simulink model "Noa_Nofusion"  (R2020b)
settings: Solver=FixedStepDiscrete  StartTime=0.0  StopTime=Inf  FixedStep=0.01  RelTol=1e-3
PostLoadFcn:
  | if any(exist('dsrtsu_mdlpostloadfcn', 'file') ~= 0), dsrtsu_mdlpostloadfcn('Execute', bdroot); end
InitFcn:
  | , if any(exist('rtifpga_mdlclblib', 'file') ~= 0), rtifpga_mdlclblib('Init', bdroot); end,
  | , if any(exist('dsmpb_private', 'file') ~= 0), dsmpb_private('dsmpb_mdlclblib', 'Init', bdroot); end,
undefined symbols (not defined in the file or in its folder): ACC_TimeGap_DecSetSwt, ACC_TimeGap_IncSetSwt, AccelPedalPosn, AccelPedalPosnVldty, AccelPedlPosnDiagc, AccPedalOverride, ACU_ShiftInProgress, ADAS_Posn_CurLane, AESSwtReq, ALC_SwtReq, BrkPedalSts, CC_ACC_CANCEL_OFFSwt, CC_ACC_CRUISE_OFFSwt, CC_ACC_DecSetSpd_SetSwt, CC_ACC_IncSetSpd_ResuSwt, CC_ACCSwtErr, CharSpd_ms, CSA_NODE, CURRENT_GEAR, CurrentGearValid, DiscIntNeverNeededParam, DrvDoorSts, DrvSBR, DrvTrqReqOvld, ECMACCInterface, ECMRespACC, ELKSwtReq, EngLimpHomeSts, EngSpd, EngState, EngState_PHEV, EngTrqMaxActSpd, EngTrqMinAct, EPS_DrvInpTrqVal_HighReslolution, EPS_FailSts, EPS_LKATorqOvrlDlvd, EPS_LKATorqOvrlDlvdVld, EPS_LKATrqOvlDlvdSts, EPS_SteerMod, EPS_TrqSnsrSts, EQ4_APPINFO, EQ4_LA_ELEM, EQ4_LA_HDR, EQ4_LAP_ELEM, EQ4_LAP_HDR, EQ4_LH_ELEM, EQ4_LH_HDR, EQ4_LRE_ELEM, EQ4_LRE_HDR, ESS_PedSwtReq, ESS_VehSwtReq, FFogLmpSts_F_Pbox, FLWheelDriveDirection, FLWheelSpd, FrntWiprSwtSts, FrntWshrSwtSts, FRWheelDriveDirection, FRWheelSpd, HazardLmpSwtSts, HCU_AccelPedalPosn_Diag ... (+151)
libraries: simulink x144, dsmpblib x33, canfdmsglib x10
(part 6 of 20)

== system Noa_Nofusion/CR_RSDS_Input/RSDS_R_Bus ==
  Enable : EnablePort
  Bus Creator : BusCreator  Inputs=9
  Bus Selector : BusSelector  OutputSignals=RSDS_R_Obj1.RSDS_R_ObjID_1 Value,RSDS_R_Obj2.RSDS_R_ObjID_2 Value,RSDS_R_Obj3.RSDS_R_ObjID_3 Value,RSDS_R_Obj4.RSDS_R_ObjID_4 Value,RSDS_R_Obj5.RSDS_R_ObjID_5 Value,RSDS_R_Obj6.RSDS_R_ObjID_6 Value
  Bus Selector1 : BusSelector  OutputSignals=RSDS_R_Obj1.RSDS_R_ObjDistX_1 Value,RSDS_R_Obj2.RSDS_R_ObjDistX_2 Value,RSDS_R_Obj3.RSDS_R_ObjDistX_3 Value,RSDS_R_Obj4.RSDS_R_ObjDistX_4 Value,RSDS_R_Obj5.RSDS_R_ObjDistX_5 Value,RSDS_R_Obj6.RSDS_R_ObjDistX_6 Value
  Bus Selector2 : BusSelector  OutputSignals=RSDS_R_Obj1.RSDS_R_ObjDistY_1 Value,RSDS_R_Obj2.RSDS_R_ObjDistY_2 Value,RSDS_R_Obj3.RSDS_R_ObjDistY_3 Value,RSDS_R_Obj4.RSDS_R_ObjDistY_4 Value,RSDS_R_Obj5.RSDS_R_ObjDistY_5 Value,RSDS_R_Obj6.RSDS_R_ObjDistY_6 Value
  Bus Selector3 : BusSelector  OutputSignals=RSDS_R_Obj1.RSDS_R_ObjRelVelX_1 Value,RSDS_R_Obj2.RSDS_R_ObjRelVelX_2 Value,RSDS_R_Obj3.RSDS_R_ObjRelVelX_3 Value,RSDS_R_Obj4.RSDS_R_ObjRelVelX_4 Value,RSDS_R_Obj5.RSDS_R_ObjRelVelX_5 Value,RSDS_R_Obj6.RSDS_R_ObjRelVelX_6 Value
  Bus Selector4 : BusSelector  OutputSignals=RSDS_R_Obj1.RSDS_R_ObjRelVelY_1 Value,RSDS_R_Obj2.RSDS_R_ObjRelVelY_2 Value,RSDS_R_Obj3.RSDS_R_ObjRelVelY_3 Value,RSDS_R_Obj4.RSDS_R_ObjRelVelY_4 Value,RSDS_R_Obj5.RSDS_R_ObjRelVelY_5 Value,RSDS_R_Obj6.RSDS_R_ObjRelVelY_6 Value
  Bus Selector5 : BusSelector  OutputSignals=RSDS_R_Obj1.RSDS_R_ObjRelAccelX_1 Value,RSDS_R_Obj2.RSDS_R_ObjRelAccelX_2 Value,RSDS_R_Obj3.RSDS_R_ObjRelAccelX_3 Value,RSDS_R_Obj4.RSDS_R_ObjRelAccelX_4 Value,RSDS_R_Obj5.RSDS_R_ObjRelAccelX_5 Value,RSDS_R_Obj6.RSDS_R_ObjRelAccelX_6 Value
  Constant : Constant  Value=uint8(4)  OutDataTypeStr=uint8
  Data Type Conversion{,1..5} (6 alike) : DataTypeConversion
  Mux{,1..5} (6 alike) : Mux  Inputs=6
  RSDS_R : MATLAB Function  TreatAsAtomicUnit=on
  RSDS_Right_Obj : dsmpblib/Data Inport  Priority=10000
      settings: SourceProductName=dSPACE Model Interface Blockset
  Terminator : Terminator
  Unit Delay : UnitDelay  SampleTime=-1  HasFrameUpgradeWarning=on
  Unit Delay1 : UnitDelay  SampleTime=-1  HasFrameUpgradeWarning=on
  RSDS_R_Obj : Outport
  wires:
  RSDS_Right_Obj/1 -> [RSDS_R_Obj]
  [RSDS_R_Obj] -> Bus Selector5/1
  Bus Selector5/3 -> Mux5/3  "<RSDS_R_ObjRelAccelX_3 Value>"
  Bus Selector3/5 -> Mux3/5  "<RSDS_R_ObjRelVelX_5 Value>"
  Unit Delay1/1 -> RSDS_R/8(ObjIDK1)
  Bus Selector5/2 -> Mux5/2  "<RSDS_R_ObjRelAccelX_2 Value>"
  Bus Selector4/3 -> Mux4/3  "<RSDS_R_ObjRelVelY_3 Value>"
  Bus Selector3/1 -> Mux3/1  "<RSDS_R_ObjRelVelX_1 Value>"
  Bus Selector2/6 -> Mux2/6  "<RSDS_R_ObjDistY_6 Value>"
  Bus Selector/6 -> Mux/6  "<RSDS_R_ObjID_6 Value>"
  Bus Selector3/2 -> Mux3/2  "<RSDS_R_ObjRelVelX_2 Value>"
  Mux5/1 -> Data Type Conversion5/1
  Bus Selector1/3 -> Mux1/3  "<RSDS_R_ObjDistX_3 Value>"
  [RSDS_R_Obj] -> Bus Selector/1
  Bus Selector1/2 -> Mux1/2  "<RSDS_R_ObjDistX_2 Value>"
  Bus Selector/2 -> Mux/2  "<RSDS_R_ObjID_2 Value>"
  Bus Selector1/5 -> Mux1/5  "<RSDS_R_ObjDistX_5 Value>"
  Bus Selector/5 -> Mux/5  "<RSDS_R_ObjID_5 Value>"
  Bus Selector2/1 -> Mux2/1  "<RSDS_R_ObjDistY_1 Value>"
  Bus Selector1/4 -> Mux1/4  "<RSDS_R_ObjDistX_4 Value>"
  Bus Selector/4 -> Mux/4  "<RSDS_R_ObjID_4 Value>"
  Mux4/1 -> Data Type Conversion4/1
  [RSDS_R_Obj] -> Bus Selector1/1
  Mux2/1 -> Data Type Conversion2/1
  Mux3/1 -> Data Type Conversion3/1
  Unit Delay/1 -> RSDS_R/9(ObjAgeK1)
  RSDS_R/10(ObjAge) -> Bus Creator/9, Unit Delay/1
  Bus Selector2/4 -> Mux2/4  "<RSDS_R_ObjDistY_4 Value>"
  Data Type Conversion/1 -> RSDS_R/2(ID)
  Bus Selector2/5 -> Mux2/5  "<RSDS_R_ObjDistY_5 Value>"
  Constant/1 -> RSDS_R/1(RadarID)
  Bus Selector3/3 -> Mux3/3  "<RSDS_R_ObjRelVelX_3 Value>"
  RSDS_R/9(ObjID) -> Unit Delay1/1, Bus Creator/8
  Data Type Conversion3/1 -> RSDS_R/5(Vx)
  RSDS_R/6(ObjAx) -> Bus Creator/5
  Bus Selector5/4 -> Mux5/4  "<RSDS_R_ObjRelAccelX_4 Value>"
  Bus Selector4/4 -> Mux4/4  "<RSDS_R_ObjRelVelY_4 Value>"
  RSDS_R/7(ObjMoveSts) -> Bus Creator/6
  Bus Creator/1 -> RSDS_R_Obj/1
  Bus Selector4/1 -> Mux4/1  "<RSDS_R_ObjRelVelY_1 Value>"
  Mux1/1 -> Data Type Conversion1/1
  RSDS_R/3(ObjDy) -> Bus Creator/2
  RSDS_R/8(ObjFusType) -> Bus Creator/7
  Bus Selector2/2 -> Mux2/2  "<RSDS_R_ObjDistY_2 Value>"
  Bus Selector1/6 -> Mux1/6  "<RSDS_R_ObjDistX_6 Value>"
  [RSDS_R_Obj] -> Bus Selector3/1
  Mux/1 -> Data Type Conversion/1
  Bus Selector1/1 -> Mux1/1  "<RSDS_R_ObjDistX_1 Value>"
  Bus Selector/3 -> Mux/3  "<RSDS_R_ObjID_3 Value>"
  Bus Selector5/1 -> Mux5/1  "<RSDS_R_ObjRelAccelX_1 Value>"
  Data Type Conversion1/1 -> RSDS_R/3(Dx)
  Bus Selector4/6 -> Mux4/6  "<RSDS_R_ObjRelVelY_6 Value>"
  Bus Selector/1 -> Mux/1  "<RSDS_R_ObjID_1 Value>"
  [RSDS_R_Obj] -> Bus Selector2/1
  RSDS_R/2(ObjDx) -> Bus Creator/1
  RSDS_R/4(ObjVx) -> Bus Creator/3
  Data Type Conversion2/1 -> RSDS_R/4(Dy)
  [RSDS_R_Obj] -> Bus Selector4/1
  Bus Selector4/2 -> Mux4/2  "<RSDS_R_ObjRelVelY_2 Value>"
  Bus Selector4/5 -> Mux4/5  "<RSDS_R_ObjRelVelY_5 Value>"
  Data Type Conversion4/1 -> RSDS_R/6(Vy)
  RSDS_R/1(P) -> Terminator/1
  Bus Selector3/6 -> Mux3/6  "<RSDS_R_ObjRelVelX_6 Value>"
  Data Type Conversion5/1 -> RSDS_R/7(Ax)
  Bus Selector5/5 -> Mux5/5  "<RSDS_R_ObjRelAccelX_5 Value>"
  Bus Selector2/3 -> Mux2/3  "<RSDS_R_ObjDistY_3 Value>"
  Bus Selector3/4 -> Mux3/4  "<RSDS_R_ObjRelVelX_4 Value>"
  RSDS_R/5(ObjVy) -> Bus Creator/4
  Bus Selector5/6 -> Mux5/6  "<RSDS_R_ObjRelAccelX_6 Value>"

== system Noa_Nofusion/Chassis1/HMA ==
  note: LightControl
  IfCANBus : Inport
  IfCALBus : Inport  Port=2
  IfDIAGBus : Inport  Port=3
  IfEQ4Bus : Inport  Port=4
  Bus Creator : BusCreator  Inputs=10
  Bus Creator1 : BusCreator  Inputs=8
  Bus Selector : BusSelector  OutputSignals=DCT_NODE.DCT5_MSG.CURRENT_GEAR,CSA_NODE.CSA1_MSG.FrntWiprSwtSts,BCM_NODE.BCM8_MSG.WiprReq_F_PBOX,PBOX_NODE.F_PBOX1_MSG.FFogLmpSts_F_Pbox,CSA_NODE.CSA1_MSG.LTurnLmpSwtSts,CSA_NODE.CSA1_MSG.RTurnLmpSwtSts,ABM_NODE.ABM2_MSG.VehYawRate,ABM_NODE.ABM2_MSG.VehLatAccel
  Bus Selector15 : BusSelector  OutputSignals=CAL_AHBC_CONFIG
  Bus Selector17 : BusSelector  OutputSignals=EQ4_HLB,EQ4_LSR,EQ4_LSV
  Bus Selector19 : BusSelector  OutputSignals=DFIM_AHBC_STS
  Bus Selector20 : BusSelector  OutputSignals=ESP_NODE.ESP_FD2_MSG.VehSpd,ESP_NODE.ESP_FD3_MSG.FLWheelDriveDirection,ESP_NODE.ESP_FD3_MSG.FRWheelDriveDirection,ESP_NODE.ESP_FD3_MSG.RLWheelDriveDirection,ESP_NODE.ESP_FD3_MSG.RRWheelDriveDirection,ESP_NODE.ESP_FD2_MSG.ABSActv,ESP_NODE.ESP_FD2_MSG.VDCActv,ESP_NODE.ESP_FD2_MSG.BTCActv,ESP_NODE.ESP_FD2_MSG.PTCActv,ESP_NODE.ESP_FD2_MSG.MSRActv
  LightControl : ModelReference  ModelNameDialog=PubIfChassisAHBC_MDL.slx  SimulationMode=Normal  ModelReferenceVersion=3.49
  IfHMABus : Outport  PortDimensions=1  BusOutputAsStruct=on
  IfADBBus : Outport  Port=2  PortDimensions=1  BusOutputAsStruct=on
  wires:
  IfDIAGBus/1 -> Bus Selector19/1
  IfCALBus/1 -> Bus Selector15/1
  IfEQ4Bus/1 -> Bus Selector17/1
  IfCANBus/1 -> Bus Selector/1, Bus Selector20/1
  LightControl/1 -> IfHMABus/1  "AHBC_HMA"
  LightControl/2 -> IfADBBus/1  "AHBC_ADB"
  Bus Selector15/1 -> LightControl/3  "<CAL_AHBC_CONFIG>"
  Bus Selector17/3 -> LightControl/6  "<EQ4_LSV>"
  Bus Selector17/2 -> LightControl/5  "<EQ4_LSR>"
  Bus Selector19/1 -> LightControl/7  "<DFIM_AHBC_STS>"
  Bus Selector20/1 -> Bus Creator/1  "<VehSpd>"
  Bus Selector20/2 -> Bus Creator/2  "<FLWheelDriveDirection>"
  Bus Selector20/3 -> Bus Creator/3  "<FRWheelDriveDirection>"
  Bus Selector20/4 -> Bus Creator/4  "<RLWheelDriveDirection>"
  Bus Selector20/5 -> Bus Creator/5  "<RRWheelDriveDirection>"
  Bus Selector20/6 -> Bus Creator/6  "<ABSActv>"
  Bus Selector20/7 -> Bus Creator/7  "<VDCActv>"
  Bus Selector20/8 -> Bus Creator/8  "<BTCActv>"
  Bus Selector20/9 -> Bus Creator/9  "<PTCActv>"
  Bus Selector20/10 -> Bus Creator/10  "<MSRActv>"
  Bus Creator/1 -> LightControl/1
  Bus Selector/1 -> Bus Creator1/1  "<CURRENT_GEAR>"
  Bus Selector/2 -> Bus Creator1/2  "<FrntWiprSwtSts>"
  Bus Selector/3 -> Bus Creator1/3  "<WiprReq_F_PBOX>"
  Bus Selector/4 -> Bus Creator1/4  "<FFogLmpSts_F_Pbox>"
  Bus Selector/5 -> Bus Creator1/5  "<LTurnLmpSwtSts>"
  Bus Selector/6 -> Bus Creator1/6  "<RTurnLmpSwtSts>"
  Bus Selector/7 -> Bus Creator1/7  "<VehYawRate>"
  Bus Selector/8 -> Bus Creator1/8  "<VehLatAccel>"
  Bus Creator1/1 -> LightControl/2
  Bus Selector17/1 -> LightControl/4  "<EQ4_HLB>"

== system Noa_Nofusion/Chassis1/HMI ==
  note: HMI
  IfVCANBus : Inport
  IfFaultTriggers : Inport  Port=2
  IfPlanbus : Inport  Port=3
  IfVSMBus : Inport  Port=4
  IfLonCtrlBus : Inport  Port=5
  IfOSMBus : Inport  Port=6
  IfAEBBus : Inport  Port=7
  IfEHRBus : Inport  Port=8
  IfDMSBus : Inport  Port=9
  LaneBus : Inport  Port=10
  RoadBus : Inport  Port=11
  In1 : Inport  Port=12
  Bus Assignment2 : BusAssignment  AssignedSignals=LSSSwtReq,ESS_PedSwtReq,ESS_VehSwtReq,AESSwtReq,IFC_SnvtySet,ADAS_Posn_CurLane,NavSpdLimValue,NavSpdLimUnit_HUT,ELKSwtReq,LCKSwtReq,LKASwtReq,LDWSwtReq
  Bus Creator : BusCreator  Inputs=10
  Bus Selector : BusSelector  OutputSignals=VSM_LON_CTRL,VSM_HMI
  Bus Selector1 : BusSelector  OutputSignals=HUT_NODE.HUT_FD1_MSG.LSSSwtReq,HUT_NODE.HUT_FD1_MSG.ESS_PedSwtReq,HUT_NODE.HUT_FD1_MSG.ESS_VehSwtReq,HUT_NODE.HUT_FD1_MSG.AESSwtReq,HUT_NODE.HUT_FD1_MSG.IFC_SnvtySet,HUT_NODE.HUT_FD1_MSG.ADAS_Posn_CurLane,HUT_NODE.HUT_FD1_MSG.NavSpdLimValue,HUT_NODE.HUT_FD1_MSG.NavSpdLimUnit_HUT,HUT_NODE.HUT_FD1_MSG.ELKSwtReq,HUT_NODE.HUT_FD1_MSG.LCKSwtReq,HUT_NODE.HUT_FD1_MSG.LKASwtReq,HUT_NODE.HUT_FD1_MSG.LDWSwtReq
  Bus Selector10 : BusSelector  OutputSignals=AEB_BRK_INFO,AEB_IPHUT_INFO
  Bus Selector11 : BusSelector  OutputSignals=RFM_TSR
  Bus Selector2 : BusSelector  OutputSignals=PLAN_HMI
  Bus Selector3 : BusSelector  Commented=on  OutputSignals=DMON_SENS_ERR
  Bus Selector4 : BusSelector  OutputSignals=LONC_CTRL_OUT
  Bus Selector6 : BusSelector  OutputSignals=TOS_ACCP0,TOS_ACCP1,TOS_ACCP2,TOS_ACCP3,TOS_ACCP4,TOS_ACCP5
  Bus Selector7 : BusSelector  OutputSignals=RFM_LINE_L1,RFM_LINE_R1,RFM_LINE_L2,RFM_LINE_R2,RFM_LINEF_LB,RFM_LINEF_RB
  Bus Selector8 : BusSelector  Commented=on  OutputSignals=EHRV2_HDR,EHRV2_HutHandshake,EHRV2_ROAD_ROI,EHRV2_ROAD_INFO
  Bus Selector9 : BusSelector  OutputSignals=DriverSts
  Constant3 : Constant  Value=0  OutDataTypeStr=Bus: VCAN_HUT_MSG_BUS
  LightControl : ModelReference  ModelNameDialog=PubIfChassisHMI_MDL.slx  SimulationMode=Normal  ModelReferenceVersion=3.97
  IfHMIBus : Outport
  wires:
  Bus Creator/1 -> IfHMIBus/1
  IfVCANBus/1 -> Bus Selector1/1
  IfFaultTriggers/1 -> Bus Selector3/1
  IfLonCtrlBus/1 -> Bus Selector4/1
  IfOSMBus/1 -> Bus Selector6/1
  LaneBus/1 -> Bus Selector7/1
  IfEHRBus/1 -> Bus Selector8/1
  IfDMSBus/1 -> Bus Selector9/1
  IfAEBBus/1 -> Bus Selector10/1
  RoadBus/1 -> Bus Selector11/1
  LightControl/1 -> Bus Creator/1  "HMI_IFC_FD2"
  LightControl/2 -> Bus Creator/2  "IFCVibrationWarning"
  LightControl/3 -> Bus Creator/3  "ESSErrSts"
  LightControl/4 -> Bus Creator/4  "AESErrSts"
  LightControl/5 -> Bus Creator/5  "HMI_ACC_FD2"
  LightControl/6 -> Bus Creator/6  "HMI_ACC_FD4"
  LightControl/7 -> Bus Creator/7  "HMI_ACC_FD1"
  LightControl/8 -> Bus Creator/8  "HMI_IFC_FD5"
  LightControl/9 -> Bus Creator/9  "HMI_IFC_FD6"
  IfVSMBus/1 -> Bus Selector/1
  Bus Selector/1 -> LightControl/1  "<VSM_LON_CTRL>"
  Bus Selector4/1 -> LightControl/27  "<LONC_CTRL_OUT>"
  Bus Selector6/1 -> LightControl/6  "<TOS_ACCP0>"
  Bus Selector6/2 -> LightControl/7  "<TOS_ACCP1>"
  Bus Selector6/3 -> LightControl/8  "<TOS_ACCP2>"
  Bus Selector6/4 -> LightControl/9  "<TOS_ACCP3>"
  Bus Selector6/5 -> LightControl/10  "<TOS_ACCP4>"
  Bus Selector6/6 -> LightControl/11  "<TOS_ACCP5>"
  Bus Selector7/1 -> LightControl/12  "<RFM_LINE_L1>"
  Bus Selector7/2 -> LightControl/13  "<RFM_LINE_R1>"
  Bus Selector7/3 -> LightControl/14  "<RFM_LINE_L2>"
  Bus Selector7/4 -> LightControl/15  "<RFM_LINE_R2>"
  Bus Selector7/5 -> LightControl/16  "<RFM_LINEF_LB>"
  Bus Selector7/6 -> LightControl/17  "<RFM_LINEF_RB>"
  Bus Selector9/1 -> LightControl/23  "<DriverSts>"
  Bus Selector10/1 -> LightControl/24  "<AEB_BRK_INFO>"
  Bus Selector10/2 -> LightControl/25  "<AEB_IPHUT_INFO>"
  Bus Selector11/1 -> LightControl/26  "<RFM_TSR>"
  Bus Selector/2 -> LightControl/2  "<VSM_HMI>"
  IfPlanbus/1 -> Bus Selector2/1
  Bus Selector2/1 -> LightControl/5  "<PLAN_HMI>"
  LightControl/10 -> Bus Creator/10  "HMI_IFC_FD3"
  Constant3/1 -> Bus Assignment2/1
  Bus Assignment2/1 -> LightControl/3
  Bus Selector1/1 -> Bus Assignment2/2  "<LSSSwtReq>"
  Bus Selector1/2 -> Bus Assignment2/3  "<ESS_PedSwtReq>"
  Bus Selector1/3 -> Bus Assignment2/4  "<ESS_VehSwtReq>"
  Bus Selector1/4 -> Bus Assignment2/5  "<AESSwtReq>"
  Bus Selector1/5 -> Bus Assignment2/6  "<IFC_SnvtySet>"
  Bus Selector1/6 -> Bus Assignment2/7  "<ADAS_Posn_CurLane>"
  Bus Selector1/7 -> Bus Assignment2/8  "<NavSpdLimValue>"
  Bus Selector1/8 -> Bus Assignment2/9  "<NavSpdLimUnit_HUT>"
  Bus Selector1/9 -> Bus Assignment2/10  "<ELKSwtReq>"
  Bus Selector1/10 -> Bus Assignment2/11  "<LCKSwtReq>"
  Bus Selector1/11 -> Bus Assignment2/12  "<LKASwtReq>"
  Bus Selector1/12 -> Bus Assignment2/13  "<LDWSwtReq>"
  In1/1 -> LightControl/28

== system Noa_Nofusion/Chassis1/Subsystem ==
  IfLatCtrlBus : Inport
  IFCFuncTrqCmdReqFlag : Inport  Port=2
  IFCTrqOvlCMdReqValue : Inport  Port=3
  IFCVirationWarning : Inport  Port=4
  Bus Assignment : BusAssignment  AssignedSignals=IFCFuncTrqCmdReqFlag,IFCTrqOvlCmdProtnValue,IFCTrqOvlCmdReqValue,IFCVibrationWarning,IFCAngCmdReqValue,IFCFuncAngCmdReqFlag,RollingCounter_IFC1,RollingCounter_IFC2
  Bus Selector : BusSelector  OutputSignals=Data
  Bus Selector1 : BusSelector  OutputSignals=LATC_IFCAngCmdReqValue,LATC_IFCFuncAngCmdReqFlag
  CAN FD Pack1 : canfdmsglib/CAN FD Pack  MsgList=(none)  MsgName=IFC_FD1  ProtocolMode=CAN FD  MsgIDType=Standard (11-bit identifier)  MsgIdentifier=299  MsgLength=64  Remote=off  BRSSwitch=on  ApplyMinMax=off  SignalInfo={ 'IFCFuncTrqCmdReqFlag', '125', '3', 'BE', 'unsigned', 'Standard', '0', '1', '0', '0', '7'; 'IFCTrqOvlCmdProtnValue', '82', '14', 'BE', 'unsigned', 'Standard', '0', '1', '0', '0', '16383'; 'IFCTrqOvlCmdReqValue', '109', '11', 'BE', 'unsigned', 'Standard', '0', '1', '-1023', '-1023', '1024'; 'IFCVibrationWarning', '104', '2', 'BE', 'unsigned', 'Standard', '0', '1', '0', '0', '3'; 'RollingCounter_IFC1', '120', '4', 'BE', 'unsigned', 'Standard', '0', '1', '0', '0', '15'; 'RollingCounter_IFC2', '184', '4', 'BE', 'unsigned', 'Standard', '0', '1', '0', '0', '15' }
      settings: SourceProductBaseCode=VN  DataFormat=manually specified signals
  CheckSum8Bclc4 : MATLAB Function  TreatAsAtomicUnit=on
  Constant : Constant  Value=0  OutDataTypeStr=Bus: IFC_FD1_MSG_BUS
  Constant4 : Constant  Value=[0x4d,0x00 0x4e 00]  OutDataTypeStr=uint8
  Constant5 : Constant  Value=1023  OutDataTypeStr=uint16
  Constant7 : Constant  Value=2^14  OutDataTypeStr=uint16
  Data Type Conversion : DataTypeConversion  OutDataTypeStr=uint16
  Data Type Conversion2 : DataTypeConversion
  Data Type Conversion3 : DataTypeConversion  OutDataTypeStr=uint16
  Gain : Gain  Gain=100
  Gain1 : Gain  Gain=2^11  OutDataTypeStr=uint32
  Gain2 : Gain  Gain=2^8  OutDataTypeStr=single
  IFC_FD1MSG1 : dsmpblib/Data Outport  Priority=-10000
      settings: SourceProductName=dSPACE Model Interface Blockset
  Rounding Function : Rounding  Operator=round
  Sum : Sum  Inputs=++++  OutDataTypeStr=uint16  RndMeth=Round
  Sum1 : Sum  Inputs=+-|  OutDataTypeStr=uint16
  rollingcounter 1 : Subsystem
  rollingcounter 2 : Subsystem
  IFC_FD1_MsgByte : Outport
  wires:
  Constant7/1 -> Sum1/1
  Data Type Conversion2/1 -> CAN FD Pack1/3
  rollingcounter 1/1(cnt) -> CAN FD Pack1/6, CAN FD Pack1/5, Gain2/1
  Constant5/1 -> Sum/3
  Constant4/1 -> CheckSum8Bclc4/2(DataID)
  IFCVirationWarning/1 -> Bus Assignment/5, CAN FD Pack1/4
  Data Type Conversion/1 -> Gain1/1
  Rounding Function/1 -> Data Type Conversion3/1, Data Type Conversion2/1
  Gain1/1 -> Sum/4
  CAN FD Pack1/1 -> Bus Selector/1
  Bus Selector/1 -> CheckSum8Bclc4/1(Data)  "<Data>"
  Gain2/1 -> Sum/1
  Data Type Conversion3/1 -> Sum/2
  Gain/1 -> Rounding Function/1
  IFCFuncTrqCmdReqFlag/1 -> Data Type Conversion/1, Bus Assignment/2, CAN FD Pack1/1
  Sum/1 -> Sum1/2
  Sum1/1 -> Bus Assignment/3, CAN FD Pack1/2
  IFCTrqOvlCMdReqValue/1 -> Bus Assignment/4, Gain/1
  CheckSum8Bclc4/1(MsgByte) -> IFC_FD1_MsgByte/1
  Constant/1 -> Bus Assignment/1
  Bus Assignment/1 -> IFC_FD1MSG1/1
  IfLatCtrlBus/1 -> Bus Selector1/1
  rollingcounter 2/1(cnt) -> Bus Assignment/9, Bus Assignment/8
  Bus Selector1/1 -> Bus Assignment/6  "<LATC_IFCAngCmdReqValue>"
  Bus Selector1/2 -> Bus Assignment/7  "<LATC_IFCFuncAngCmdReqFlag>"

== system Noa_Nofusion/Chassis1/Subsystem1 ==
  In13 : Inport
  <PLAN_Longctrl_DecelToStopReq> : Inport  Port=2
  Bus Assignment : BusAssignment  AssignedSignals=ACC_CRInterface,ActualTargetSpeed,Longctrl_DecelToStopReq,Longctrl_Decel_Req,Longctrl_Decel_ReqValue,Longctrl_DrvOFF_Req,Longctrl_EngTrqReq,Longctrl_EngTrqReqActive,Longctrl_FuelCutOffPrevn,Longctrl_ModSts,Longctrl_ParkShiftReq,Longctrl_VehHldReq,Longctrl_HCUTrqReq,Longctrl_HCUTrqReqActive,HWP_TgtAccel_L2
  Bus Selector18 : BusSelector  OutputSignals=HMI.HMI_ACC_FD1.ACC_CRInterface,HMI.HMI_ACC_FD1.ActualTargetSpeed,signal2.LONC_CTRL_OUT.Longctrl_Decel_Req,signal2.LONC_CTRL_OUT.Longctrl_Decel_ReqValue,HMI.HMI_ACC_FD1.Longctrl_DrvOFF_Req,signal2.LONC_CTRL_OUT.Longctrl_EngTrqReq,signal2.LONC_CTRL_OUT.Longctrl_EngTrqReqActive,HMI.HMI_ACC_FD1.Longctrl_FuelCutOffPrevn,HMI.HMI_ACC_FD1.Longctrl_ModSts,HMI.HMI_ACC_FD1.Longctrl_ParkShiftReq,HMI.HMI_ACC_FD1.Longctrl_VehHldReq,signal2.LONC_Hybrid_CTRL_OUT.Longctrl_HCUTrqReq,signal2.LONC_Hybrid_CTRL_OUT.Longctrl_HCUTrqReqActive
  Constant : Constant  Value=0  OutDataTypeStr=Bus: ACC_FD1_MSG_BUS
  Constant1 : Constant  Value=255
  Data Type Conversion : DataTypeConversion
  Out9 : Outport
  wires:
  Constant/1 -> Bus Assignment/1
  Bus Assignment/1 -> Out9/1
  In13/1 -> Bus Selector18/1
  Bus Selector18/1 -> Bus Assignment/2  "<ACC_CRInterface>"
  Bus Selector18/2 -> Bus Assignment/3  "<ActualTargetSpeed>"
  Bus Selector18/3 -> Bus Assignment/5  "<Longctrl_Decel_Req>"
  Bus Selector18/4 -> Bus Assignment/6  "<Longctrl_Decel_ReqValue>"
  Bus Selector18/5 -> Bus Assignment/7  "<Longctrl_DrvOFF_Req>"
  Bus Selector18/6 -> Bus Assignment/8  "<Longctrl_EngTrqReq>"
  Bus Selector18/7 -> Bus Assignment/9  "<Longctrl_EngTrqReqActive>"
  Bus Selector18/8 -> Bus Assignment/10  "<Longctrl_FuelCutOffPrevn>"
  Bus Selector18/9 -> Bus Assignment/11  "<Longctrl_ModSts>"
  Bus Selector18/10 -> Bus Assignment/12  "<Longctrl_ParkShiftReq>"
  Bus Selector18/11 -> Bus Assignment/13  "<Longctrl_VehHldReq>"
  Constant1/1 -> Data Type Conversion/1
  Data Type Conversion/1 -> Bus Assignment/16
  <PLAN_Longctrl_DecelToStopReq>/1 -> Bus Assignment/4
  Bus Selector18/12 -> Bus Assignment/14  "<Longctrl_HCUTrqReq>"
  Bus Selector18/13 -> Bus Assignment/15  "<Longctrl_HCUTrqReqActive>"

== system Noa_Nofusion/Chassis1/rollingcounter 1 ==
  Constant7 : Constant  OutDataTypeStr=Inherit: Inherit via back propagation
  Constant8 : Constant  Value=14  OutDataTypeStr=Inherit: Inherit via back propagation
  Constant9 : Constant  Value=0  OutDataTypeStr=Inherit: Inherit via back propagation
  Relational Operator : RelationalOperator  Operator=>  OutDataTypeStr=boolean  RndMeth=Nearest
  Sum : Sum  Inputs=|++
  Switch : Switch  Criteria=u2 ~= 0  Threshold=1
  Unit Delay : UnitDelay  SampleTime=-1  HasFrameUpgradeWarning=on
  cnt : Outport
  wires:
  Switch/1 -> Unit Delay/1, cnt/1
  Relational Operator/1 -> Switch/2
  Constant7/1 -> Sum/1
  Unit Delay/1 -> Sum/2
  Constant8/1 -> Relational Operator/2
  Sum/1 -> Relational Operator/1, Switch/3
  Constant9/1 -> Switch/1

== system Noa_Nofusion/Chassis1/rollingcounter 2 ==
  Constant7 : Constant  OutDataTypeStr=Inherit: Inherit via back propagation
  Constant8 : Constant  Value=14  OutDataTypeStr=Inherit: Inherit via back propagation
  Constant9 : Constant  Value=0  OutDataTypeStr=Inherit: Inherit via back propagation
  Relational Operator : RelationalOperator  Operator=>  OutDataTypeStr=boolean  RndMeth=Nearest
  Sum : Sum  Inputs=|++
  Switch : Switch  Criteria=u2 ~= 0  Threshold=1
  Unit Delay : UnitDelay  SampleTime=-1  HasFrameUpgradeWarning=on
  cnt : Outport
  wires:
  Constant9/1 -> Switch/1
  Sum/1 -> Switch/3, Relational Operator/1
  Constant8/1 -> Relational Operator/2
  Unit Delay/1 -> Sum/2
  Constant7/1 -> Sum/1
  Relational Operator/1 -> Switch/2
  Switch/1 -> cnt/1, Unit Delay/1

== system Noa_Nofusion/Chassis1/rollingcounter 3 ==
  Constant7 : Constant  OutDataTypeStr=Inherit: Inherit via back propagation
  Constant8 : Constant  Value=14  OutDataTypeStr=Inherit: Inherit via back propagation
  Constant9 : Constant  Value=0  OutDataTypeStr=Inherit: Inherit via back propagation
  Relational Operator : RelationalOperator  Operator=>  OutDataTypeStr=boolean  RndMeth=Nearest
  Sum : Sum  Inputs=|++
  Switch : Switch  Criteria=u2 ~= 0  Threshold=1
  Unit Delay : UnitDelay  SampleTime=-1  HasFrameUpgradeWarning=on
  cnt : Outport
  wires:
  Switch/1 -> Unit Delay/1, cnt/1
  Relational Operator/1 -> Switch/2
  Constant7/1 -> Sum/1
  Unit Delay/1 -> Sum/2
  Constant8/1 -> Relational Operator/2
  Sum/1 -> Relational Operator/1, Switch/3
  Constant9/1 -> Switch/1

== system Noa_Nofusion/Chassis1/rollingcounter 4 ==
  Constant7 : Constant  OutDataTypeStr=Inherit: Inherit via back propagation
  Constant8 : Constant  Value=14  OutDataTypeStr=Inherit: Inherit via back propagation
  Constant9 : Constant  Value=0  OutDataTypeStr=Inherit: Inherit via back propagation
  Relational Operator : RelationalOperator  Operator=>  OutDataTypeStr=boolean  RndMeth=Nearest
  Sum : Sum  Inputs=|++
  Switch : Switch  Criteria=u2 ~= 0  Threshold=1
  Unit Delay : UnitDelay  SampleTime=-1  HasFrameUpgradeWarning=on
  cnt : Outport
  wires:
  Constant9/1 -> Switch/1
  Sum/1 -> Switch/3, Relational Operator/1
  Constant8/1 -> Relational Operator/2
  Unit Delay/1 -> Sum/2
  Constant7/1 -> Sum/1
  Relational Operator/1 -> Switch/2
  Switch/1 -> cnt/1, Unit Delay/1

== system Noa_Nofusion/Common/CAL ==
  CAL_VSM_CONFIG : Outport  OutDataTypeStr=Bus: CAL_VSM_CONFIG_BUS  PortDimensions=1  BusOutputAsStruct=on
  CAL_AEB_CONFIG : Outport  Port=2  OutDataTypeStr=Bus: CAL_AEB_CONFIG_BUS  PortDimensions=1  BusOutputAsStruct=on
  NvMReadWriteU8 : Outport  Port=3  OutDataTypeStr=uint8  PortDimensions=1  BusOutputAsStruct=on
  CAL_AHBC_CONFIG : Outport  Port=4  OutDataTypeStr=Bus: CAL_AHBC_CONFIG_BUS  PortDimensions=1  BusOutputAsStruct=on

== system Noa_Nofusion/Common/Subsystem1 ==
  In1 : Inport
  Bus Creator5 : BusCreator  Inputs=11
  Bus Selector2 : BusSelector  OutputSignals=HUT_NODE.HUT_FD1_MSG.ADAS_Posn_Offset,HUT_NODE.HUT_FD1_MSG.ADAS_Posn_MsgTye,HUT_NODE.HUT_FD1_MSG.ADAS_Posn_Pathldx,HUT_NODE.HUT_FD1_MSG.ADAS_Posn_CycCnt,HUT_NODE.HUT_FD1_MSG.ADAS_Posn_Age,HUT_NODE.HUT_FD1_MSG.ADAS_Posn_PosProbb,HUT_NODE.HUT_FD1_MSG.ADAS_Posn_Idx,HUT_NODE.HUT_FD1_MSG.ADAS_Posn_Spd,HUT_NODE.HUT_FD1_MSG.ADAS_Posn_CurLane,HUT_NODE.HUT_FD1_MSG.ADAS_Posn_PosConfdc,HUT_NODE.HUT_FD1_MSG.ADAS_Posn_Rehead
  EHRV2_VCAN_POSN : Outport
  wires:
  Bus Selector2/4 -> Bus Creator5/4  "<ADAS_Posn_CycCnt>"
  Bus Selector2/7 -> Bus Creator5/7  "<ADAS_Posn_Idx>"
  Bus Selector2/6 -> Bus Creator5/6  "<ADAS_Posn_PosProbb>"
  Bus Selector2/9 -> Bus Creator5/9  "<ADAS_Posn_CurLane>"
  Bus Selector2/11 -> Bus Creator5/11  "<ADAS_Posn_Rehead>"
  Bus Selector2/8 -> Bus Creator5/8  "<ADAS_Posn_Spd>"
  Bus Selector2/2 -> Bus Creator5/2  "<ADAS_Posn_MsgTye>"
  Bus Selector2/3 -> Bus Creator5/3  "<ADAS_Posn_Pathldx>"
  Bus Selector2/5 -> Bus Creator5/5  "<ADAS_Posn_Age>"
  Bus Selector2/1 -> Bus Creator5/1  "<ADAS_Posn_Offset>"
  Bus Selector2/10 -> Bus Creator5/10  "<ADAS_Posn_PosConfdc>"
  Bus Creator5/1 -> EHRV2_VCAN_POSN/1
  In1/1 -> Bus Selector2/1

== system Noa_Nofusion/Common/Subsystem2 ==
  In1 : Inport
  Bus Creator5 : BusCreator  Inputs=12
  Bus Selector6 : BusSelector  OutputSignals=HUT_NODE.HUT21_MSG.ADAS_ProfShort_Offset,HUT_NODE.HUT21_MSG.ADAS_ProfShort_MsgTyp,HUT_NODE.HUT21_MSG.ADAS_ProfShort_PathIdx,HUT_NODE.HUT21_MSG.ADAS_ProfShort_CycCnt,HUT_NODE.HUT21_MSG.ADAS_ProfShort_Update,HUT_NODE.HUT21_MSG.ADAS_ProfShort_Retr,HUT_NODE.HUT21_MSG.ADAS_ProfShort_CtrlPoint,HUT_NODE.HUT21_MSG.ADAS_ProfShort_ProfTyp,HUT_NODE.HUT21_MSG.ADAS_ProfShort_Dist1,HUT_NODE.HUT21_MSG.ADAS_ProfShort_AccurClass,HUT_NODE.HUT21_MSG.ADAS_ProfShort_Value0,HUT_NODE.HUT21_MSG.ADAS_ProfShort_Value1
  EHRV2_VCAN_PROFSHORT : Outport
  wires:
  Bus Selector6/7 -> Bus Creator5/7  "<ADAS_ProfShort_CtrlPoint>"
  Bus Selector6/4 -> Bus Creator5/4  "<ADAS_ProfShort_CycCnt>"
  Bus Selector6/6 -> Bus Creator5/6  "<ADAS_ProfShort_Retr>"
  Bus Selector6/9 -> Bus Creator5/9  "<ADAS_ProfShort_Dist1>"
  Bus Selector6/5 -> Bus Creator5/5  "<ADAS_ProfShort_Update>"
  Bus Selector6/12 -> Bus Creator5/12  "<ADAS_ProfShort_Value1>"
  Bus Selector6/11 -> Bus Creator5/11  "<ADAS_ProfShort_Value0>"
  Bus Selector6/10 -> Bus Creator5/10  "<ADAS_ProfShort_AccurClass>"
  Bus Selector6/8 -> Bus Creator5/8  "<ADAS_ProfShort_ProfTyp>"
  Bus Creator5/1 -> EHRV2_VCAN_PROFSHORT/1
  Bus Selector6/3 -> Bus Creator5/3  "<ADAS_ProfShort_PathIdx>"
  Bus Selector6/1 -> Bus Creator5/1  "<ADAS_ProfShort_Offset>"
  Bus Selector6/2 -> Bus Creator5/2  "<ADAS_ProfShort_MsgTyp>"
  In1/1 -> Bus Selector6/1

== system Noa_Nofusion/Common/Subsystem3 ==
  In1 : Inport
  Bus Creator7 : BusCreator  Inputs=17
  Bus Selector4 : BusSelector  OutputSignals=HUT_NODE.HUT23_MSG.ADAS_Stub_Offset,HUT_NODE.HUT23_MSG.ADAS_Stub_MsgTyp,HUT_NODE.HUT23_MSG.ADAS_Stub_PathIdx,HUT_NODE.HUT23_MSG.ADAS_Stub_CycCnt,HUT_NODE.HUT23_MSG.ADAS_Stub_Update,HUT_NODE.HUT23_MSG.ADAS_Stub_Retr,HUT_NODE.HUT23_MSG.ADAS_Stub_StubPathIdx,HUT_NODE.HUT23_MSG.ADAS_Stub_FuncRoadClass,HUT_NODE.HUT23_MSG.ADAS_Stub_RelProbb,HUT_NODE.HUT23_MSG.ADAS_Stub_FormOfWay,HUT_NODE.HUT23_MSG.ADAS_Stub_CmplxInsct,HUT_NODE.HUT23_MSG.ADAS_Stub_PartOfCalcRoute,HUT_NODE.HUT23_MSG.ADAS_Stub_TurnAngl,HUT_NODE.HUT23_MSG.ADAS_Stub_NumOfLaneDrvDir,HUT_NODE.HUT23_MSG.ADAS_Stub_NumOfLaneOppDir,HUT_NODE.HUT23_MSG.ADAS_Stub_RtOfWay,HUT_NODE.HUT23_MSG.ADAS_Stub_LastStub
  EHRV2_VCAN_STUB : Outport
  wires:
  Bus Selector4/8 -> Bus Creator7/8  "<ADAS_Stub_FuncRoadClass>"
  Bus Selector4/10 -> Bus Creator7/10  "<ADAS_Stub_FormOfWay>"
  Bus Selector4/2 -> Bus Creator7/2  "<ADAS_Stub_MsgTyp>"
  Bus Selector4/4 -> Bus Creator7/4  "<ADAS_Stub_CycCnt>"
  Bus Selector4/5 -> Bus Creator7/5  "<ADAS_Stub_Update>"
  Bus Selector4/3 -> Bus Creator7/3  "<ADAS_Stub_PathIdx>"
  Bus Selector4/1 -> Bus Creator7/1  "<ADAS_Stub_Offset>"
  Bus Selector4/7 -> Bus Creator7/7  "<ADAS_Stub_StubPathIdx>"
  Bus Selector4/6 -> Bus Creator7/6  "<ADAS_Stub_Retr>"
  Bus Selector4/11 -> Bus Creator7/11  "<ADAS_Stub_CmplxInsct>"
  Bus Selector4/9 -> Bus Creator7/9  "<ADAS_Stub_RelProbb>"
  Bus Selector4/12 -> Bus Creator7/12  "<ADAS_Stub_PartOfCalcRoute>"
  Bus Selector4/15 -> Bus Creator7/15  "<ADAS_Stub_NumOfLaneOppDir>"
  Bus Selector4/16 -> Bus Creator7/16  "<ADAS_Stub_RtOfWay>"
  Bus Selector4/17 -> Bus Creator7/17  "<ADAS_Stub_LastStub>"
  Bus Selector4/13 -> Bus Creator7/13  "<ADAS_Stub_TurnAngl>"
  In1/1 -> Bus Selector4/1
  Bus Creator7/1 -> EHRV2_VCAN_STUB/1
  Bus Selector4/14 -> Bus Creator7/14  "<ADAS_Stub_NumOfLaneDrvDir>"

== system Noa_Nofusion/Common/Subsystem4 ==
  In1 : Inport
  Bus Creator6 : BusCreator  Inputs=9
  Bus Selector7 : BusSelector  OutputSignals=HUT_NODE.HUT20_MSG.ADAS_ProfLong_Offset,HUT_NODE.HUT20_MSG.ADAS_ProfLong_MsgTyp,HUT_NODE.HUT20_MSG.ADAS_ProfLong_PathIdx,HUT_NODE.HUT20_MSG.ADAS_ProfLong_CycCnt,HUT_NODE.HUT20_MSG.ADAS_ProfLong_Update,HUT_NODE.HUT20_MSG.ADAS_ProfLong_Retr,HUT_NODE.HUT20_MSG.ADAS_ProfLong_CtrlPoint,HUT_NODE.HUT20_MSG.ADAS_ProfLong_ProfTyp,HUT_NODE.HUT20_MSG.ADAS_ProfLong_Value
  EHRV2_VCAN_PROFLONG : Outport
  wires:
  Bus Selector7/9 -> Bus Creator6/9  "<ADAS_ProfLong_Value>"
  Bus Selector7/3 -> Bus Creator6/3  "<ADAS_ProfLong_PathIdx>"
  Bus Selector7/2 -> Bus Creator6/2  "<ADAS_ProfLong_MsgTyp>"
  Bus Selector7/8 -> Bus Creator6/8  "<ADAS_ProfLong_ProfTyp>"
  Bus Selector7/7 -> Bus Creator6/7  "<ADAS_ProfLong_CtrlPoint>"
  Bus Selector7/5 -> Bus Creator6/5  "<ADAS_ProfLong_Update>"
  Bus Creator6/1 -> EHRV2_VCAN_PROFLONG/1
  Bus Selector7/4 -> Bus Creator6/4  "<ADAS_ProfLong_CycCnt>"
  Bus Selector7/1 -> Bus Creator6/1  "<ADAS_ProfLong_Offset>"
  Bus Selector7/6 -> Bus Creator6/6  "<ADAS_ProfLong_Retr>"
  In1/1 -> Bus Selector7/1

== system Noa_Nofusion/Common/Subsystem5 ==
  In1 : Inport
  Bus Creator5 : BusCreator  Inputs=19
  Bus Selector5 : BusSelector  OutputSignals=HUT_NODE.HUT22_MSG.ADAS_Seg_Offset,HUT_NODE.HUT22_MSG.ADAS_Seg_MsgTyp,HUT_NODE.HUT22_MSG.ADAS_Seg_PathIdx,HUT_NODE.HUT22_MSG.ADAS_Seg_CycCnt,HUT_NODE.HUT22_MSG.ADAS_Seg_Update,HUT_NODE.HUT22_MSG.ADAS_Seg_Retr,HUT_NODE.HUT22_MSG.ADAS_Seg_BuildUpArea,HUT_NODE.HUT22_MSG.ADAS_Seg_Brdg,HUT_NODE.HUT22_MSG.ADAS_Seg_Tunnel,HUT_NODE.HUT22_MSG.ADAS_Seg_FuncRoadClass,HUT_NODE.HUT22_MSG.ADAS_Seg_RelProbb,HUT_NODE.HUT22_MSG.ADAS_Seg_FormOfWay,HUT_NODE.HUT22_MSG.ADAS_Seg_CmplxInsct,HUT_NODE.HUT22_MSG.ADAS_Seg_PartOfCalcRoute,HUT_NODE.HUT22_MSG.ADAS_Seg_EffSpdLmtTyp,HUT_NODE.HUT22_MSG.ADAS_Seg_EffSpdLmt,HUT_NODE.HUT22_MSG.ADAS_Seg_NumOfLaneDrvDir,HUT_NODE.HUT22_MSG.ADAS_Seg_NumOfLaneOppDir,HUT_NODE.HUT22_MSG.ADAS_Seg_DivideRoad
  EHRV2_VCAN_SEG : Outport
  wires:
  Bus Selector5/6 -> Bus Creator5/6  "<ADAS_Seg_Retr>"
  Bus Selector5/7 -> Bus Creator5/7  "<ADAS_Seg_BuildUpArea>"
  Bus Selector5/14 -> Bus Creator5/14  "<ADAS_Seg_PartOfCalcRoute>"
  Bus Selector5/8 -> Bus Creator5/8  "<ADAS_Seg_Brdg>"
  Bus Selector5/4 -> Bus Creator5/4  "<ADAS_Seg_CycCnt>"
  Bus Selector5/1 -> Bus Creator5/1  "<ADAS_Seg_Offset>"
  Bus Selector5/15 -> Bus Creator5/15  "<ADAS_Seg_EffSpdLmtTyp>"
  Bus Selector5/16 -> Bus Creator5/16  "<ADAS_Seg_EffSpdLmt>"
  Bus Selector5/5 -> Bus Creator5/5  "<ADAS_Seg_Update>"
  Bus Selector5/13 -> Bus Creator5/13  "<ADAS_Seg_CmplxInsct>"
  Bus Selector5/17 -> Bus Creator5/17  "<ADAS_Seg_NumOfLaneDrvDir>"
  Bus Creator5/1 -> EHRV2_VCAN_SEG/1
  Bus Selector5/18 -> Bus Creator5/18  "<ADAS_Seg_NumOfLaneOppDir>"
  Bus Selector5/2 -> Bus Creator5/2  "<ADAS_Seg_MsgTyp>"
  Bus Selector5/11 -> Bus Creator5/11  "<ADAS_Seg_RelProbb>"
  Bus Selector5/3 -> Bus Creator5/3  "<ADAS_Seg_PathIdx>"
  Bus Selector5/19 -> Bus Creator5/19  "<ADAS_Seg_DivideRoad>"
  Bus Selector5/12 -> Bus Creator5/12  "<ADAS_Seg_FormOfWay>"
  Bus Selector5/10 -> Bus Creator5/10  "<ADAS_Seg_FuncRoadClass>"
  Bus Selector5/9 -> Bus Creator5/9  "<ADAS_Seg_Tunnel>"
  In1/1 -> Bus Selector5/1

== system Noa_Nofusion/Common/Subsystem6 ==
  In1 : Inport
  Bus Creator5 : BusCreator  Inputs=13
  Bus Selector3 : BusSelector  OutputSignals=HUT_NODE.HUT19_MSG.ADAS_Meta_CountryCode,HUT_NODE.HUT19_MSG.ADAS_Meta_MapProvider,HUT_NODE.HUT19_MSG.ADAS_Meta_MsgTyp,HUT_NODE.HUT19_MSG.ADAS_Meta_HwVer,HUT_NODE.HUT19_MSG.ADAS_Meta_ProtVer_MinorSub,HUT_NODE.HUT19_MSG.ADAS_Meta_ProtVer_Major,HUT_NODE.HUT19_MSG.ADAS_Meta_CycCnt,HUT_NODE.HUT19_MSG.ADAS_Meta_RegionCode,HUT_NODE.HUT19_MSG.ADAS_Meta_DrvSide,HUT_NODE.HUT19_MSG.ADAS_Meta_MapVerYear,HUT_NODE.HUT19_MSG.ADAS_Meta_MapVerQtr,HUT_NODE.HUT19_MSG.ADAS_Meta_ProtVer_Minor,HUT_NODE.HUT19_MSG.ADAS_Meta_SpdUnits
  EHRV2_VCAN_META : Outport
  wires:
  Bus Selector3/1 -> Bus Creator5/1  "<ADAS_Meta_CountryCode>"
  Bus Selector3/10 -> Bus Creator5/10  "<ADAS_Meta_MapVerYear>"
  Bus Selector3/4 -> Bus Creator5/4  "<ADAS_Meta_HwVer>"
  Bus Selector3/2 -> Bus Creator5/2  "<ADAS_Meta_MapProvider>"
  Bus Selector3/5 -> Bus Creator5/5  "<ADAS_Meta_ProtVer_MinorSub>"
  Bus Selector3/7 -> Bus Creator5/7  "<ADAS_Meta_CycCnt>"
  Bus Selector3/8 -> Bus Creator5/8  "<ADAS_Meta_RegionCode>"
  Bus Selector3/9 -> Bus Creator5/9  "<ADAS_Meta_DrvSide>"
  Bus Selector3/3 -> Bus Creator5/3  "<ADAS_Meta_MsgTyp>"
  Bus Selector3/6 -> Bus Creator5/6  "<ADAS_Meta_ProtVer_Major>"
  Bus Selector3/11 -> Bus Creator5/11  "<ADAS_Meta_MapVerQtr>"
  Bus Selector3/13 -> Bus Creator5/13  "<ADAS_Meta_SpdUnits>"
  Bus Selector3/12 -> Bus Creator5/12  "<ADAS_Meta_ProtVer_Minor>"
  In1/1 -> Bus Selector3/1
  Bus Creator5/1 -> EHRV2_VCAN_META/1

== system Noa_Nofusion/Common/Subsystem7 ==
  DMSSts : Inport  OutDataTypeStr=uint8  PortDimensions=1  Interpolate=off  BusOutputAsStruct=on
  HeadDetn : Inport  Port=2  OutDataTypeStr=boolean  PortDimensions=1  Interpolate=off  BusOutputAsStruct=on
  DistrctnLvl_ACC : Inport  Port=3  OutDataTypeStr=uint8  PortDimensions=1  Interpolate=off  BusOutputAsStruct=on
  DistrctnLvlQlty_ACC : Inport  Port=4  OutDataTypeStr=uint8  PortDimensions=1  Interpolate=off  BusOutputAsStruct=on
  DrowsnsLvl_ACC : Inport  Port=5  OutDataTypeStr=uint8  PortDimensions=1  Interpolate=off  BusOutputAsStruct=on
  DS : Subsystem  Commented=on
  DMS_DistractnSts : Outport
  DMS_DrowsnsSts : Outport  Port=2
  DMS_DriverSts : Outport  Port=3
  wires:
  DrowsnsLvl_ACC/1 -> DS/5(canDrowsnsLevel)
  DistrctnLvlQlty_ACC/1 -> DS/4(canDistrctnQlty)
  DistrctnLvl_ACC/1 -> DS/3(canDistrctnLevel)
  DMSSts/1 -> DS/1(canDMSSts)
  HeadDetn/1 -> DS/2(canHeadDetn)
  DS/3(DriverSts) -> DMS_DriverSts/1  "DMS_DriverSts"
  DS/2(DrowsnsSts) -> DMS_DrowsnsSts/1  "DMS_DrowsnsSts"
  DS/1(DistractnSts) -> DMS_DistractnSts/1  "DMS_DistractnSts"

== system Noa_Nofusion/Control1/Subsystem ==
  In1 : Inport
  Bus Assignment3 : BusAssignment  AssignedSignals=NetEngTrq,MaxEngTrqNorm,EngTrqMinAct,EngTrqMaxActSpd,EngSpd
  Bus Selector14 : BusSelector  OutputSignals=ECM_NODE.ECM_FD1_MSG.NetEngTrq,ECM_NODE.ECM_FD3_MSG.MaxEngTrqNorm,ECM_NODE.ECM_FD1_MSG.EngTrqMinAct,ECM_NODE.ECM_FD1_MSG.EngTrqMaxActSpd,ECM_NODE.ECM_FD1_MSG.EngSpd
  Constant2 : Constant  Value=0  OutDataTypeStr=Bus: VCAN_ECM_MSG_BUS
  Out1 : Outport
  wires:
  Bus Selector14/3 -> Bus Assignment3/4  "<EngTrqMinAct>"
  Bus Assignment3/1 -> Out1/1
  Bus Selector14/5 -> Bus Assignment3/6  "<EngSpd>"
  Bus Selector14/4 -> Bus Assignment3/5  "<EngTrqMaxActSpd>"
  Constant2/1 -> Bus Assignment3/1
  In1/1 -> Bus Selector14/1
  Bus Selector14/2 -> Bus Assignment3/3  "<MaxEngTrqNorm>"
  Bus Selector14/1 -> Bus Assignment3/2  "<NetEngTrq>"

== system Noa_Nofusion/EQ4_Lane_Pack1/For Each Subsystem1 ==
  In1 : Inport  Partition=on  PartitionDimension=1  PartitionWidth=1  PartitionOffset=0
  Bus Assignment4 : BusAssignment  AssignedSignals=LH_CRC,LH_Is_Triggered_SDM_Type,LH_Is_Triggered_SDM_Model,LH_Track_ID,LH_Age,LH_Confidence,Reserved_3,LH_Prediction_Reason,LH_Availability_State,LH_Color,LH_Color_Confidence,LH_Lanemark_Type,LH_DLM_Type,LH_DECEL_Type,Reserved_4,LH_Lanemark_Type_Conf,LH_Side,LH_Crossing,LH_Marker_Width,LH_Marker_Width_STD,Reserved_5,LH_Dash_Average_Length,LH_Dash_Average_Gap,LH_Is_Multi_Clothoid,Reserved_6,LH_Line_First_C0,LH_Line_First_C1,LH_Line_First_C2,LH_Line_First_C3,LH_First_VR_Start,LH_First_VR_End,Reserved_7,LH_First_Measured_VR_End,LH_Second_Measured_VR_End,Reserved_8,LH_Line_Second_C0,LH_Line_Second_C1,LH_Line_Second_C2,LH_Line_Second_C3,LH_Second_VR_Start,LH_Second_VR_End,LH_Buffer_C3
  Bus Selector : BusSelector  OutputSignals=LH_CRC,LH_Is_Triggered_SDM_Type,LH_Is_Triggered_SDM_Model,LH_Track_ID,LH_Age,LH_Confidence,Reserved_3,LH_Prediction_Reason,LH_Availability_State,LH_Color,LH_Color_Confidence,LH_Lanemark_Type,LH_DLM_Type,LH_DECEL_Type,Reserved_4,LH_Lanemark_Type_Conf,LH_Side,LH_Crossing,LH_Marker_Width,LH_Marker_Width_STD,Reserved_5,LH_Dash_Average_Length,LH_Dash_Average_Gap,LH_Is_Multi_Clothoid,Reserved_6,LH_Line_First_C0,LH_Line_First_C1,LH_Line_First_C2,LH_Line_First_C3,LH_First_VR_Start,LH_First_VR_End,Reserved_7,LH_First_Measured_VR_End,LH_Second_Measured_VR_End,Reserved_8,LH_Line_Second_C0,LH_Line_Second_C1,LH_Line_Second_C2,LH_Line_Second_C3,LH_Second_VR_Start,LH_Second_VR_End,LH_Buffer_C3
  Constant4 : Constant  Value=0  OutDataTypeStr=Bus: EQ4_LH_ELEM_BUS
  For Each : ForEach  DisableCoverage=on
  Out1 : Outport  ConcatenationDimension=1
  wires:
  Constant4/1 -> Bus Assignment4/1
  In1/1 -> Bus Selector/1
  Bus Assignment4/1 -> Out1/1
  Bus Selector/1 -> Bus Assignment4/2  "<LH_CRC>"
  Bus Selector/2 -> Bus Assignment4/3  "<LH_Is_Triggered_SDM_Type>"
  Bus Selector/3 -> Bus Assignment4/4  "<LH_Is_Triggered_SDM_Model>"
  Bus Selector/4 -> Bus Assignment4/5  "<LH_Track_ID>"
  Bus Selector/5 -> Bus Assignment4/6  "<LH_Age>"
  Bus Selector/6 -> Bus Assignment4/7  "<LH_Confidence>"
  Bus Selector/7 -> Bus Assignment4/8  "<Reserved_3>"
  Bus Selector/8 -> Bus Assignment4/9  "<LH_Prediction_Reason>"
  Bus Selector/9 -> Bus Assignment4/10  "<LH_Availability_State>"
  Bus Selector/10 -> Bus Assignment4/11  "<LH_Color>"
  Bus Selector/11 -> Bus Assignment4/12  "<LH_Color_Confidence>"
  Bus Selector/12 -> Bus Assignment4/13  "<LH_Lanemark_Type>"
  Bus Selector/13 -> Bus Assignment4/14  "<LH_DLM_Type>"
  Bus Selector/14 -> Bus Assignment4/15  "<LH_DECEL_Type>"
  Bus Selector/15 -> Bus Assignment4/16  "<Reserved_4>"
  Bus Selector/16 -> Bus Assignment4/17  "<LH_Lanemark_Type_Conf>"
  Bus Selector/17 -> Bus Assignment4/18  "<LH_Side>"
  Bus Selector/18 -> Bus Assignment4/19  "<LH_Crossing>"
  Bus Selector/19 -> Bus Assignment4/20  "<LH_Marker_Width>"
  Bus Selector/20 -> Bus Assignment4/21  "<LH_Marker_Width_STD>"
  Bus Selector/21 -> Bus Assignment4/22  "<Reserved_5>"
  Bus Selector/22 -> Bus Assignment4/23  "<LH_Dash_Average_Length>"
  Bus Selector/23 -> Bus Assignment4/24  "<LH_Dash_Average_Gap>"
  Bus Selector/24 -> Bus Assignment4/25  "<LH_Is_Multi_Clothoid>"
  Bus Selector/25 -> Bus Assignment4/26  "<Reserved_6>"
  Bus Selector/26 -> Bus Assignment4/27  "<LH_Line_First_C0>"
  Bus Selector/27 -> Bus Assignment4/28  "<LH_Line_First_C1>"
  Bus Selector/28 -> Bus Assignment4/29  "<LH_Line_First_C2>"
  Bus Selector/29 -> Bus Assignment4/30  "<LH_Line_First_C3>"
  Bus Selector/30 -> Bus Assignment4/31  "<LH_First_VR_Start>"
  Bus Selector/31 -> Bus Assignment4/32  "<LH_First_VR_End>"
  Bus Selector/32 -> Bus Assignment4/33  "<Reserved_7>"
  Bus Selector/33 -> Bus Assignment4/34  "<LH_First_Measured_VR_End>"
  Bus Selector/34 -> Bus Assignment4/35  "<LH_Second_Measured_VR_End>"
  Bus Selector/35 -> Bus Assignment4/36  "<Reserved_8>"
  Bus Selector/36 -> Bus Assignment4/37  "<LH_Line_Second_C0>"
  Bus Selector/37 -> Bus Assignment4/38  "<LH_Line_Second_C1>"
  Bus Selector/38 -> Bus Assignment4/39  "<LH_Line_Second_C2>"
  Bus Selector/39 -> Bus Assignment4/40  "<LH_Line_Second_C3>"
  Bus Selector/40 -> Bus Assignment4/41  "<LH_Second_VR_Start>"
  Bus Selector/41 -> Bus Assignment4/42  "<LH_Second_VR_End>"
  Bus Selector/42 -> Bus Assignment4/43  "<LH_Buffer_C3>"

== system Noa_Nofusion/EQ4_Lane_Pack1/For Each Subsystem2 ==
  In1 : Inport  Partition=on  PartitionDimension=1  PartitionWidth=1  PartitionOffset=0
  Bus Assignment4 : BusAssignment  AssignedSignals=LRE_ID,LRE_Age,LRE_Confidence,LRE_Type,Reserved_2,LRE_Prediction_Reason,LRE_Availability_State,LRE_Height,LRE_Height_STD,Reserved_3,LRE_View_Range_Start,LRE_View_Range_End,Reserved_4,LRE_Measured_VR_End,LRE_Side,LRE_Is_Triggered_SDM_Model,Reserved_5,LRE_Line_C3,LRE_Line_C2,LRE_Line_C1,LRE_Line_C0,LRE_Detection_Source,Reserved_6
  Bus Selector : BusSelector  OutputSignals=LRE_ID,LRE_Age,LRE_Confidence,LRE_Type,Reserved_2,LRE_Prediction_Reason,LRE_Availability_State,LRE_Height,LRE_Height_STD,Reserved_3,LRE_View_Range_Start,LRE_View_Range_End,Reserved_4,LRE_Measured_VR_End,LRE_Side,LRE_Is_Triggered_SDM_Model,Reserved_5,LRE_Line_C3,LRE_Line_C2,LRE_Line_C1,LRE_Line_C0,LRE_Detection_Source,Reserved_6
  Constant4 : Constant  Value=0  OutDataTypeStr=Bus: EQ4_LRE_ELEM_BUS
  For Each : ForEach  DisableCoverage=on
  Out1 : Outport  ConcatenationDimension=1
  wires:
  Bus Assignment4/1 -> Out1/1
  In1/1 -> Bus Selector/1
  Constant4/1 -> Bus Assignment4/1
  Bus Selector/1 -> Bus Assignment4/2  "<LRE_ID>"
  Bus Selector/2 -> Bus Assignment4/3  "<LRE_Age>"
  Bus Selector/3 -> Bus Assignment4/4  "<LRE_Confidence>"
  Bus Selector/4 -> Bus Assignment4/5  "<LRE_Type>"
  Bus Selector/5 -> Bus Assignment4/6  "<Reserved_2>"
  Bus Selector/6 -> Bus Assignment4/7  "<LRE_Prediction_Reason>"
  Bus Selector/7 -> Bus Assignment4/8  "<LRE_Availability_State>"
  Bus Selector/8 -> Bus Assignment4/9  "<LRE_Height>"
  Bus Selector/9 -> Bus Assignment4/10  "<LRE_Height_STD>"
  Bus Selector/10 -> Bus Assignment4/11  "<Reserved_3>"
  Bus Selector/11 -> Bus Assignment4/12  "<LRE_View_Range_Start>"
  Bus Selector/12 -> Bus Assignment4/13  "<LRE_View_Range_End>"
  Bus Selector/13 -> Bus Assignment4/14  "<Reserved_4>"
  Bus Selector/14 -> Bus Assignment4/15  "<LRE_Measured_VR_End>"
  Bus Selector/15 -> Bus Assignment4/16  "<LRE_Side>"
  Bus Selector/16 -> Bus Assignment4/17  "<LRE_Is_Triggered_SDM_Model>"
  Bus Selector/17 -> Bus Assignment4/18  "<Reserved_5>"
  Bus Selector/18 -> Bus Assignment4/19  "<LRE_Line_C3>"
  Bus Selector/19 -> Bus Assignment4/20  "<LRE_Line_C2>"
  Bus Selector/20 -> Bus Assignment4/21  "<LRE_Line_C1>"
  Bus Selector/21 -> Bus Assignment4/22  "<LRE_Line_C0>"
  Bus Selector/22 -> Bus Assignment4/23  "<LRE_Detection_Source>"
  Bus Selector/23 -> Bus Assignment4/24  "<Reserved_6>"

== system Noa_Nofusion/EQ4_Lane_Pack1/For Each Subsystem3 ==
  In1 : Inport  Partition=on  PartitionDimension=1  PartitionWidth=1  PartitionOffset=0
  Bus Assignment4 : BusAssignment  AssignedSignals=LA_Lane_Track_ID,LA_Age,LA_Confidence,LA_Color,LA_Color_Conf,LA_Prediction_Reason,LA_Availability_State,LA_View_Range_Start,Reserved_2,LA_View_Range_End,LA_Measured_VR_End,Reserved_3,LA_Lanemark_Type,LA_DLM_Type,LA_Lanemark_Type_Conf,LA_Line_Side,LA_Marker_Width,Reserved_4,LA_Marker_Width_STD,Reserved_5,LA_Line_C3,LA_Line_C2,LA_Line_C1,LA_Line_C0,LH_Buffer_C1,Reserved_6
  Bus Selector : BusSelector  OutputSignals=LA_Lane_Track_ID,LA_Age,LA_Confidence,LA_Color,LA_Color_Conf,LA_Prediction_Reason,LA_Availability_State,LA_View_Range_Start,Reserved_2,LA_View_Range_End,LA_Measured_VR_End,Reserved_3,LA_Lanemark_Type,LA_DLM_Type,LA_Lanemark_Type_Conf,LA_Line_Side,LA_Marker_Width,Reserved_4,LA_Marker_Width_STD,Reserved_5,LA_Line_C3,LA_Line_C2,LA_Line_C1,LA_Line_C0,LH_Buffer_C1,Reserved_6
  Constant4 : Constant  Value=0  OutDataTypeStr=Bus: EQ4_LA_ELEM_BUS
  For Each : ForEach  DisableCoverage=on
  Out1 : Outport  ConcatenationDimension=1
  wires:
  Bus Assignment4/1 -> Out1/1
  In1/1 -> Bus Selector/1
  Constant4/1 -> Bus Assignment4/1
  Bus Selector/1 -> Bus Assignment4/2  "<LA_Lane_Track_ID>"
  Bus Selector/2 -> Bus Assignment4/3  "<LA_Age>"
  Bus Selector/3 -> Bus Assignment4/4  "<LA_Confidence>"
  Bus Selector/4 -> Bus Assignment4/5  "<LA_Color>"
  Bus Selector/5 -> Bus Assignment4/6  "<LA_Color_Conf>"
  Bus Selector/6 -> Bus Assignment4/7  "<LA_Prediction_Reason>"
  Bus Selector/7 -> Bus Assignment4/8  "<LA_Availability_State>"
  Bus Selector/8 -> Bus Assignment4/9  "<LA_View_Range_Start>"
  Bus Selector/9 -> Bus Assignment4/10  "<Reserved_2>"
  Bus Selector/10 -> Bus Assignment4/11  "<LA_View_Range_End>"
  Bus Selector/11 -> Bus Assignment4/12  "<LA_Measured_VR_End>"
  Bus Selector/12 -> Bus Assignment4/13  "<Reserved_3>"
  Bus Selector/13 -> Bus Assignment4/14  "<LA_Lanemark_Type>"
  Bus Selector/14 -> Bus Assignment4/15  "<LA_DLM_Type>"
  Bus Selector/15 -> Bus Assignment4/16  "<LA_Lanemark_Type_Conf>"
  Bus Selector/16 -> Bus Assignment4/17  "<LA_Line_Side>"
  Bus Selector/17 -> Bus Assignment4/18  "<LA_Marker_Width>"
  Bus Selector/18 -> Bus Assignment4/19  "<Reserved_4>"
  Bus Selector/19 -> Bus Assignment4/20  "<LA_Marker_Width_STD>"
  Bus Selector/20 -> Bus Assignment4/21  "<Reserved_5>"
  Bus Selector/21 -> Bus Assignment4/22  "<LA_Line_C3>"
  Bus Selector/22 -> Bus Assignment4/23  "<LA_Line_C2>"
  Bus Selector/23 -> Bus Assignment4/24  "<LA_Line_C1>"
  Bus Selector/24 -> Bus Assignment4/25  "<LA_Line_C0>"
  Bus Selector/25 -> Bus Assignment4/26  "<LH_Buffer_C1>"
  Bus Selector/26 -> Bus Assignment4/27  "<Reserved_6>"

== system Noa_Nofusion/EQ4_Lane_Pack1/For Each Subsystem4 ==
  In1 : Inport  Partition=on  PartitionDimension=1  PartitionWidth=1  PartitionOffset=0
  Bus Assignment4 : BusAssignment  AssignedSignals=LAP_INTP_ID,LAP_INTP_Distance_Age,LAP_INTP_Confidence,LAP_INTP_Is_Valid,LAP_INTP_Type,LAP_INTP_Is_Start,Reserved_4,LAP_INTP_Lat_Distance,LAP_INTP_Long_Distance,Reserved_5,LAP_Buffer_C1,LAP_Buffer_C2,Reserved_6
  Bus Selector : BusSelector  OutputSignals=LAP_INTP_ID,LAP_INTP_Distance_Age,LAP_INTP_Confidence,LAP_INTP_Is_Valid,LAP_INTP_Type,LAP_INTP_Is_Start,Reserved_4,LAP_INTP_Lat_Distance,LAP_INTP_Long_Distance,Reserved_5,LAP_Buffer_C1,LAP_Buffer_C2,Reserved_6,Reserved_7
  Constant4 : Constant  Value=0  OutDataTypeStr=Bus: EQ4_LAP_ELEM_BUS
  For Each : ForEach  DisableCoverage=on
  Out1 : Outport  ConcatenationDimension=1
  wires:
  Constant4/1 -> Bus Assignment4/1
  In1/1 -> Bus Selector/1
  Bus Assignment4/1 -> Out1/1
  Bus Selector/1 -> Bus Assignment4/2  "<LAP_INTP_ID>"
  Bus Selector/2 -> Bus Assignment4/3  "<LAP_INTP_Distance_Age>"
  Bus Selector/3 -> Bus Assignment4/4  "<LAP_INTP_Confidence>"
  Bus Selector/4 -> Bus Assignment4/5  "<LAP_INTP_Is_Valid>"
  Bus Selector/5 -> Bus Assignment4/6  "<LAP_INTP_Type>"
  Bus Selector/6 -> Bus Assignment4/7  "<LAP_INTP_Is_Start>"
  Bus Selector/7 -> Bus Assignment4/8  "<Reserved_4>"
  Bus Selector/8 -> Bus Assignment4/9  "<LAP_INTP_Lat_Distance>"
  Bus Selector/9 -> Bus Assignment4/10  "<LAP_INTP_Long_Distance>"
  Bus Selector/10 -> Bus Assignment4/11  "<Reserved_5>"
  Bus Selector/11 -> Bus Assignment4/12  "<LAP_Buffer_C1>"
  Bus Selector/12 -> Bus Assignment4/13  "<LAP_Buffer_C2>"
  Bus Selector/13 -> Bus Assignment4/14  "<Reserved_6>"

== system Noa_Nofusion/LPV/ABM_Pack ==
  In1 : Inport
  Bus Assignment2 : BusAssignment  AssignedSignals=DrvSBR,PassSBR,VehLgtAccel,VehLatAccel,VehYawRate
  Bus Selector14 : BusSelector  OutputSignals=ABM_NODE.ABM1_MSG.DrvSBR,ABM_NODE.ABM1_MSG.PassSBR,ABM_NODE.ABM2_MSG.VehLgtAccel,ABM_NODE.ABM2_MSG.VehLatAccel,ABM_NODE.ABM2_MSG.VehYawRate
  Constant3 : Constant  Value=0  OutDataTypeStr=Bus: VCAN_ABM_MSG_BUS
  VSM_VCAN_ABM : Outport
  wires:
  Bus Assignment2/1 -> VSM_VCAN_ABM/1
  In1/1 -> Bus Selector14/1
  Constant3/1 -> Bus Assignment2/1
  Bus Selector14/5 -> Bus Assignment2/6  "<VehYawRate>"
  Bus Selector14/4 -> Bus Assignment2/5  "<VehLatAccel>"
  Bus Selector14/3 -> Bus Assignment2/4  "<VehLgtAccel>"
  Bus Selector14/2 -> Bus Assignment2/3  "<PassSBR>"
  Bus Selector14/1 -> Bus Assignment2/2  "<DrvSBR>"

== system Noa_Nofusion/LPV/BCM_Pack ==
  In1 : Inport
  Bus Assignment2 : BusAssignment  AssignedSignals=WiprReq_F_PBOX,DrvDoorSts,PassengerDoorSts,WindshldWiprActvSts,HazardLmpSwtSts,KL30BRelaySts
  Bus Selector10 : BusSelector  OutputSignals=BCM_NODE.BCM8_MSG.WiprReq_F_PBOX,BCM_NODE.BCM1_MSG.DrvDoorSts,BCM_NODE.BCM1_MSG.PassengerDoorSts,BCM_NODE.BCM1_MSG.WindshldWiprActvSts,BCM_NODE.BCM3_MSG.HazardLmpSwtSts,BCM_NODE.BCM8_MSG.KL30BRelaySts
  Constant3 : Constant  Value=0  OutDataTypeStr=Bus: VCAN_BCM_MSG_BUS
  VSM_VCAN_BCM : Outport
  wires:
  In1/1 -> Bus Selector10/1
  Bus Assignment2/1 -> VSM_VCAN_BCM/1
  Constant3/1 -> Bus Assignment2/1
  Bus Selector10/3 -> Bus Assignment2/4  "<PassengerDoorSts>"
  Bus Selector10/4 -> Bus Assignment2/5  "<WindshldWiprActvSts>"
  Bus Selector10/2 -> Bus Assignment2/3  "<DrvDoorSts>"
  Bus Selector10/5 -> Bus Assignment2/6  "<HazardLmpSwtSts>"
  Bus Selector10/1 -> Bus Assignment2/2  "<WiprReq_F_PBOX>"
  Bus Selector10/6 -> Bus Assignment2/7  "<KL30BRelaySts>"
